simulink model "WMmodel"  (R2025a)
settings: Solver=daessc  StartTime=0.0  StopTime=7200  MaxStep=.5  RelTol=1e-3  AbsTol=1e-3
PreLoadFcn:
  | WMmodel_ini
  | Control_Ts=2;
values from neighbouring files (symbols this model uses):
  inletPipeDia = 0.025    [WMmodel_ini.m]
  motorRatedSpeed = 1250    [WMmodel_ini.m]
  motorRotorInertia = 1e-3    (= 0.001)    [WMmodel_ini.m]
  outerDrumLen = 1    [WMmodel_ini.m]
  outerDrumMaxFill = 50    [WMmodel_ini.m]
  outletPipeDia = 0.025    [WMmodel_ini.m]
  valveSpoolPosMax = 0.01    [WMmodel_ini.m]
libraries: fl_lib x17, nesl_utility x9, SimscapeFluids_lib x7, sdl_lib x1, ee_lib x1
CloseFcn:
  | try,close(h1_sscv_washing_machine_fault_analysis),end
  | clear h1_sscv_washing_machine_fault_analysis
  | 
  | clear outerDrumLiqLevel_ini outerDrumArea
  | clear outerDrumLen outerDrumMaxFill
  | clear outletPipeEffLen outletPipeDia
  | clear inletPipeEffLen inletPipeDia
  | clear valveSpoolPosMax valveSpoolTravel
  | clear valveFaultTime pumpShaftSpeed
  | clear motorPhase motorNumPolePair motorRatedMechPower
  | clear motorRatedSpeed motorRatedRMScurr motorEff
  | clear motorRotorInertia motorRotorDamping
  | clear pumpCapacity pumpHead pumpBrakePower
  | clear Control_Ts
  | clear simlog_sscv_washing_machine_fault_analysis tout
Description:
  | Washing Machine Fault Analysis
settings Model: Creator=The MathWorks, Inc.  LastModifiedBy=DR53SF
settings SolverCC: AutoScaleAbsTol=off  MaxConsecutiveMinStep=5  ZeroCrossAlgorithm=Adaptive  AlgebraicLoopSolver=TrustRegion  MaxZcPerStep=1.0
settings DataIOCC: ReturnWorkspaceOutputs=off
settings OptimizationCC: ReuseModelBlockBuffer=off
settings DebuggingCC: IgnoredZcDiagnostic=none  UnconnectedInputMsg=warning  UnconnectedOutputMsg=warning  UnconnectedLineMsg=warning  SymbolicDimsDataTypeCodeGenerationDiagnostic=none
settings ModelReferenceCC: EnableRefExpFcnMdlSchedulingChecks=on
settings SFSimCC: CustomCodeUndefinedFunction=UseInterfaceOnly
settings RTWCC: GPUComputeCapability=3.5  DLArmComputeVersion=19.05
settings SimscapeCC: SimscapeNominalValues="[{\"value\":\"1\",\"unit\":\"A\"},{\"value\":\"1\",\"unit\":\"bar\"},{\"value\":\"1\",\"unit\":\"cm^2\"},{\"value\":\"1\",\"unit\":\"cm^3/s\"},{\"value\":\"1\",\"unit\":\"kJ/kg\"},{\"value\":\"1\",\"unit\":\"kW\"},{\"value\":\"1\",\"unit\":\"l\"},{\"value\":\"1\",\"unit\":\"N\"},{\"value\":\"1\",\"unit\":\"N*m\"},{\"value\":\"1\",\"unit\":\"V\"},{\"value\":\"1e-2\",\"unit\":\"m\"}]"  SimscapeLogType=all  SimscapeLogSimulationStatistics=on  SimscapeLogName=simlog_sscv_washing_machine_fault_analysis  SimscapeLogDataHistory=100000.0

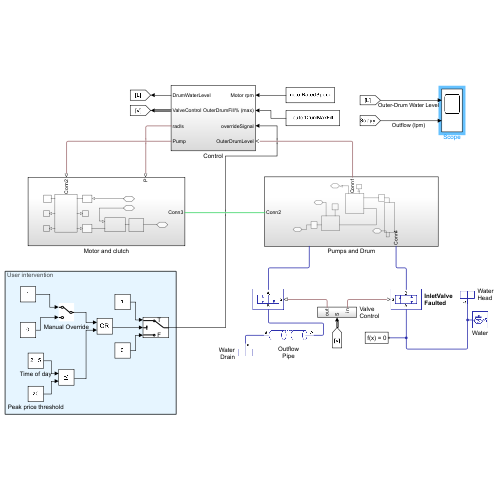
[thumbnail: Simulink's stored preview of the top-level diagram]
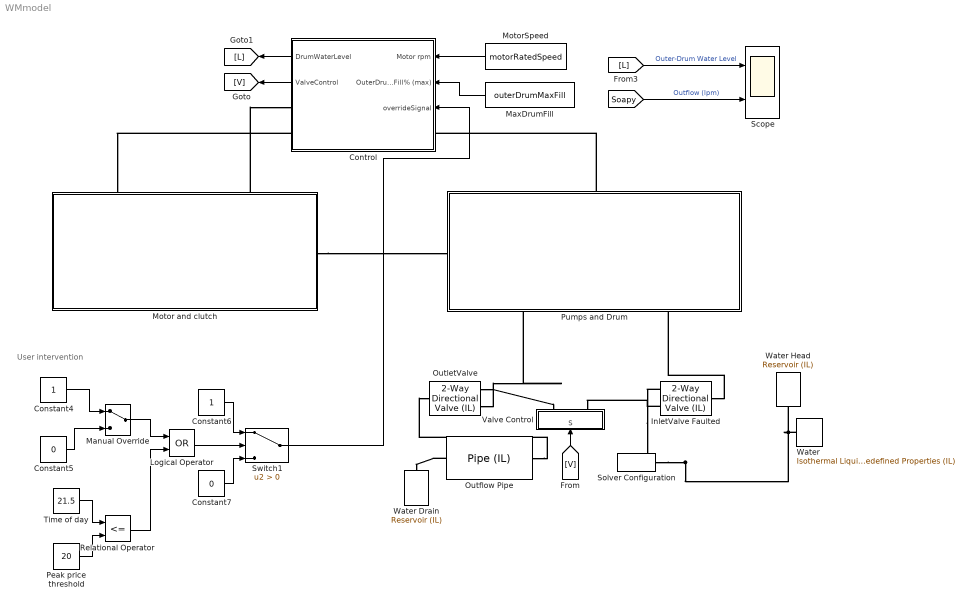
== system WMmodel ==
  note: User intervention
  Constant4 : Constant
  Constant5 : Constant  Value=0
  Constant6 : Constant
  Constant7 : Constant  Value=0
  Control : Subsystem
  InletValve Faulted : SimscapeFluids_lib/Isothermal Liquid/Valves & Orifices/Directional Control Valves/2-Way Directional Valve (IL)  valve_spec=fluids.isothermal_liquid.valves_orifices.directional_control_valves.enum.directional_valve_spec.linear  S_max=valveSpoolPosMax m  del_S_max=valveSpoolTravel m  area_max=(pi/4)*inletPipeDia^2 m^2  area_leak=1e-10 m^2  del_S_TLU=[0, .002, .004, .007, .017] m  orifice_area_TLU=[1e-09, 2.0352e-07, 4.0736e-05, .00011438, .00034356] m^2  del_S_vol_flow_TLU=[0, .002, .004, .007, .017] m  p_diff_TLU=[.003, .05, .7] MPa  vol_flow_TLU=1e-3 * [1.7e-05, 2e-05, 2.6e-05; .0035, .0045, .0053; .7, .9, 1.06; 1.96, 2.5, 3; 6, 7.7, 9.13] m^3/s  Cd=0.64  Re_c=150  smoothing_factor=0.01  pressure_recovery=simscape.enum.onoff.off  area=inf m^2
      settings: InternalSimscapePortConfiguration="{\"Bottom\":[{\"id\":\"B\",\"label\":\"B\",\"type\":\"foundation.isothermal_liquid.isothermal_liquid\"}],\"Left\":[{\"id\":\"S\",\"label\":\"S\",\"type\":\"input\"}],\"Right\":[],\"Top\":[{\"id\":\"A\",\"label\":\"A\",\"type\":\"foundation.isothermal_liquid.isothermal_liquid\"}]}"
  Logical Operator : Logic  Operator=OR  AllPortsSameDT=off  OutDataTypeStr=boolean
  Manual Override : ManualSwitch
  MaxDrumFill : Constant  Value=outerDrumMaxFill  SampleTime=Control_Ts
  Motor and clutch : Subsystem
      settings: PortSchema="{\"entries\":[{\"content\":{\"sides\":[{\"content\":{},\"type\":\"ConnectorPlacement.EquallySpacedRectSide\",\"uuid\":\"2cb3139e-4bf3-4635-b004-e0199a90a34f\"},{\"content\":{\"connectorIds\":[\"RConn1\"],\"side\":\"RIGHT\"},\"type\":\"ConnectorPlacement.EquallySpacedRectSide\",\"uuid\":\"0fa1d438-5e01-49a5-a846-ce380dc8e568\"},{\"content\":{\"connectorIds\":[\"LConn1\",\"LConn2\"],\"side\":\"TOP\"},\"type\":\"ConnectorPlacement.EquallySpacedRectSide\",\"uuid\":\"2360d654-7a91-4e53-9178-c914f2ea5ea3\"}]},\"type\":\"ConnectorPlacement.EquallySpacedConnector\",\"uuid\":\"18350a3b-7253-46c1-a86d-3a50888f0ef8\"}],\"packageUris\":[\"http://schema.mathworks.com/mf0/Connector/R2020b\"],\"version\":\"1.0\"}"
  MotorSpeed : Constant  Value=motorRatedSpeed  SampleTime=Control_Ts
  Outflow Pipe : SimscapeFluids_lib/Isothermal Liquid/Pipes & Fittings/Pipe (IL)  dynamic_compressibility=simscape.enum.onoff.off  inertia=simscape.enum.onoff.off  num_segments=1  pipe_length=outletPipeEffLen m  cross_section_geometry=fluids.isothermal_liquid.pipes_fittings.enum.cross_section_geometry.circular  pipe_diameter=outletPipeDia m  pipe_inner_diameter=0.05 m  pipe_outer_diameter=0.1 m  pipe_width=0.1 m  pipe_height=0.1 m  pipe_major_axis=0.1 m  pipe_minor_axis=0.05 m  pipe_side=0.1 m  pipe_angle=30 deg  pipe_area=0.01 m^2  Dh=0.1128 m  elevation_spec=foundation.enum.constant_variable.constant  elevation_gain=0 m  gravity_spec=foundation.enum.constant_variable.constant  g=9.81 m/s^2  pressure_loss_spec=fluids.isothermal_liquid.pipes_fittings.enum.pressure_loss_spec.haaland  mdot_nominal=[.1, 1] kg/s  p_diff_nominal=[.001, .01] MPa  mdot_threshold=1e-6 kg/s  local_pressure_loss_spec=fluids.isothermal_liquid.pipes_fittings.enum.local_loss_spec.aggregate_length  length_add=1 m  loss_coefficient=0.1  roughness_spec=fluids.isothermal_liquid.pipes_fittings.enum.roughness_spec.commercial_pipe  roughness=15e-6 m  Re_friction_TLU=[400, 1000, 1500, 3000, 4000, 6000, 10000, 20000, 40000, 60000, 100000, 100000000]  friction_factor_TLU=[.264, .112, .071, .0417, .0387, .0268, .025, .0232, .0226, .022, .0214, .0214]  Re_lam=2000  Re_tur=4000  shape_factor=64  pipe_wall_spec=fluids.isothermal_liquid.pipes_fittings.enum.wall_spec.rigid  vol_expansion_spec=fluids.isothermal_liquid.pipes_fittings.enum.vol_expansion_spec.area  area_pressure_gain=1e-6 m^2/MPa  static_pressure_TLU=[.1, 1] MPa  area_pressure_gain_TLU=[1e-05, 1.1e-05] m^2  material_behavior_spec=fluids.isothermal_liquid.pipes_fittings.enum.PipeMaterialBehavior.Linear  diameter_pressure_gain=1e-6 m/MPa  wall_thickness=0.05 m  elastic_modulus=69 GPa  stress_TLU=[276, 310] MPa  strain_TLU=[.004, .02]  stress_assert_action=simscape.enum.assert.action.none  stress_max=400 MPa  poisson_ratio=0.33  wall_time_constant=0.01 s  p0=0.101325 MPa  mdot0=0 kg/s
      settings: InternalSimscapePortConfiguration="{\"Bottom\":[],\"Left\":[{\"id\":\"A\",\"label\":\"A\",\"type\":\"foundation.isothermal_liquid.isothermal_liquid\"}],\"Right\":[{\"id\":\"B\",\"label\":\"B\",\"type\":\"foundation.isothermal_liquid.isothermal_liquid\"}],\"Top\":[]}"
  OutletValve : SimscapeFluids_lib/Isothermal Liquid/Valves & Orifices/Directional Control Valves/2-Way Directional Valve (IL)  valve_spec=fluids.isothermal_liquid.valves_orifices.directional_control_valves.enum.directional_valve_spec.linear  S_max=valveSpoolPosMax m  del_S_max=valveSpoolTravel m  area_max=(pi/4)*outletPipeDia^2 m^2  area_leak=1e-10 m^2  del_S_TLU=[0, .002, .004, .007, .017] m  orifice_area_TLU=[1e-09, 2.0352e-07, 4.0736e-05, .00011438, .00034356] m^2  del_S_vol_flow_TLU=[0, .002, .004, .007, .017] m  p_diff_TLU=[.003, .05, .7] MPa  vol_flow_TLU=1e-3 * [1.7e-05, 2e-05, 2.6e-05; .0035, .0045, .0053; .7, .9, 1.06; 1.96, 2.5, 3; 6, 7.7, 9.13] m^3/s  Cd=0.64  Re_c=150  smoothing_factor=0.01  pressure_recovery=simscape.enum.onoff.off  area=inf m^2
      settings: InternalSimscapePortConfiguration="{\"Bottom\":[{\"id\":\"B\",\"label\":\"B\",\"type\":\"foundation.isothermal_liquid.isothermal_liquid\"}],\"Left\":[{\"id\":\"S\",\"label\":\"S\",\"type\":\"input\"}],\"Right\":[],\"Top\":[{\"id\":\"A\",\"label\":\"A\",\"type\":\"foundation.isothermal_liquid.isothermal_liquid\"}]}"
  Peak price threshold : Constant  Value=20
  Pumps and Drum : Subsystem
      settings: PortSchema="{\"entries\":[{\"content\":{\"sides\":[{\"content\":{\"connectorIds\":[\"LConn1\"]},\"type\":\"ConnectorPlacement.EquallySpacedRectSide\",\"uuid\":\"b631024b-b03a-4ba5-88ab-f74a9126b18e\"},{\"content\":{\"side\":\"RIGHT\"},\"type\":\"ConnectorPlacement.EquallySpacedRectSide\",\"uuid\":\"3fd644d5-b563-41d8-9687-2eeaabd5b41f\"},{\"content\":{\"connectorIds\":[\"LConn2\"],\"side\":\"TOP\"},\"type\":\"ConnectorPlacement.EquallySpacedRectSide\",\"uuid\":\"584c2d8d-6c1b-48df-bb3f-7aaa8986bf0f\"},{\"content\":{\"connectorIds\":[\"RConn1\",\"RConn2\"],\"side\":\"BOTTOM\"},\"type\":\"ConnectorPlacement.EquallySpacedRectSide\",\"uuid\":\"c0a6f7af-5a5a-4250-abd1-d4c5b47363d7\"}]},\"type\":\"ConnectorPlacement.EquallySpacedConnector\",\"uuid\":\"531ac8a9-248c-40a4-8545-6bc81e2e4632\"}],\"packageUris\":[\"http://schema.mathworks.com/mf0/Connector/R2020b\"],\"version\":\"1.0\"}"
  Relational Operator : RelationalOperator  Operator=<=  OutDataTypeStr=boolean  RndMeth=Simplest  InputSameDT=off
  Scope : Scope  NumInputPorts=2
      settings: ActiveDisplayYMinimum=-0.01080540819902244  ActiveDisplayYMaximum=0.56392239287112012  YLabel=Level (m)
  Solver Configuration : nesl_utility/Solver Configuration  PhysicalDomain=network_engine_domain  SubClassName=solver  LeftPortType=input  RightPortType=generic  Tones=[]  Harmonics=[]  SimulateNoise=off  Profile=off  UseLocalSampling=off  EnableSwitchedLinearOptims=on  FrequencyDomain=off  UseCCode=off  RelTol=0.001  AbsTol=1e-06  MinStep=1e-09  ToWorkspace=off  RevertToSquareIcSolve=off  NumHomotopyIterations=100  PhasorMode=off  PhasorModeNumHarmonics=1  ConsistencySolver=NEWTON_FTOL  IndexReductionMethod=DerivativeReplacement  DoDC=off  ResidualTolerance=1e-9  ConsistencyTolSource=GLOBAL  ConsistencyAbsTol=0.001  ConsistencyRelTol=0.001  ConsistencyTolFactor=0.001  UseLocalSolver=off  LocalSolverChoice=NE_BACKWARD_EULER_ADVANCER  ResolveIndetEquations=on  FunctionEvalNumThread=1  LocalSolverSampleTime=.5  DoFixedCost=off  MaxNonlinIter=50  MaxModeIter=2  ComputeImpulses=off  ImpulseIterations=2  LinearAlgebra=auto  LinearAlgebraNumThread=0  EquationFormulation=NE_TIME_EF  DelaysMemoryBudget=1024  AutomaticFiltering=off  FilteringTimeConstant=0.001  PartitionStorageMethod=AS_NEEDED  PartitionMemoryBudget=1024  PartitionMethod=FAST  MultibodyUseLocalSolver=off  MultibodyLocalSolverChoice=ODE1  MultibodyLocalSolverSampleTime=0.001
  Switch1 : Switch  Criteria=u2 > Threshold  SaturateOnIntegerOverflow=off  InputSameDT=off
  Time of day : Constant  Value=21.5
  Valve Control : Subsystem
  Water : SimscapeFluids_lib/Isothermal Liquid/Utilities/Isothermal Liquid Predefined Properties (IL)  fluid_list=fluids.isothermal_liquid.utilities.enum.isothermal_liquid_fluid_list.water  concentration_param_EG=fluids.isothermal_liquid.utilities.enum.isothermal_liquid_concentration.volume_fraction  concentration_param_PG=fluids.isothermal_liquid.utilities.enum.isothermal_liquid_concentration.volume_fraction  c_mass_SW=3.5e-3  c_mass_EG=0.1  c_mass_PG=0.1  c_mass_GL=0.1  c_vol_EG=0.1  c_vol_PG=0.1  beta_L_atm_EG=2.1791 GPa  beta_L_atm_PG=2.1791 GPa  beta_L_atm_GL=2.1791 GPa  p_min_EG=0.01 MPa  p_min_PG=0.01 MPa  p_min_GL=0.01 MPa  T=293.15 K  derate_coeff=1  p_atm=0.101325 MPa  properties_range_check=simscape.enum.assert.action.error  air_fraction=0  polytropic_index=1.0  rho_g_atm=1.225 kg/m^3  air_dissolution_model=simscape.enum.onoff.off  p_crit=3 MPa
      settings: InternalSimscapePortConfiguration="{\"Bottom\":[],\"Left\":[],\"Right\":[{\"id\":\"A\",\"label\":\"\",\"type\":\"foundation.isothermal_liquid.isothermal_liquid\"}],\"Top\":[]}"
  Water Drain : fl_lib/Isothermal Liquid/Elements/Reservoir (IL)  reservoir_type=foundation.enum.constant_controlled.constant  pressure_spec=foundation.enum.pressure_spec.atmospheric  reservoir_pressure=0.101325 MPa
  Water Head : fl_lib/Isothermal Liquid/Elements/Reservoir (IL)  reservoir_type=foundation.enum.constant_controlled.constant  pressure_spec=foundation.enum.pressure_spec.specified  reservoir_pressure=.11 MPa
  wires:
  MaxDrumFill/1 -> Control/2(OuterDrumFill% (max))
  [Soapy] -> Scope/2  "Outflow (lpm)"
  Control/2(ValveControl) -> [V]
  [V] -> Valve Control/1(S)
  MotorSpeed/1 -> Control/1(Motor rpm)
  Control/1(DrumWaterLevel) -> [L]
  [L] -> Scope/1  "Outer-Drum Water Level"
  Constant5/1 -> Manual Override/2
  Constant6/1 -> Switch1/1
  Relational Operator/1 -> Logical Operator/2
  Time of day/1 -> Relational Operator/1
  Constant7/1 -> Switch1/3
  Logical Operator/1 -> Switch1/2
  Manual Override/1 -> Logical Operator/1
  Constant4/1 -> Manual Override/1
  Peak price threshold/1 -> Relational Operator/2
  Switch1/1 -> Control/3(overrideSignal)
  connections:
  Water/RConn1 -- InletValve Faulted/LConn2 -- Solver Configuration/RConn1 -- Water Head/LConn1
  OutletValve/LConn1 -- Valve Control/RConn1
  Outflow Pipe/LConn1 -- OutletValve/RConn1
  Outflow Pipe/RConn1 -- Water Drain/LConn1
  InletValve Faulted/LConn1 -- Valve Control/RConn2
  Motor and clutch/LConn2 -- Control/RConn1
  Control/RConn2 -- Motor and clutch/LConn1
  Pumps and Drum/LConn2 -- Control/LConn1
  Motor and clutch/RConn1 -- Pumps and Drum/LConn1
  OutletValve/LConn2 -- Pumps and Drum/RConn1
  InletValve Faulted/RConn1 -- Pumps and Drum/RConn2

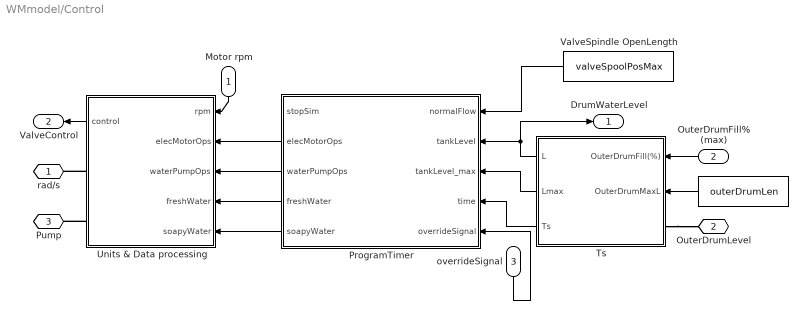
== system WMmodel/Control ==
  Motor rpm : Inport
  OuterDrumFill% (max) : Inport  Port=2
  overrideSignal : Inport  Port=3
  "  " : Constant  Value=outerDrumLen  SampleTime=Control_Ts
  ProgramTimer : MATLAB Function  TreatAsAtomicUnit=on
  Ts : Subsystem
  Units & Data processing : Subsystem
  ValveSpindle OpenLength : Constant  Value=valveSpoolPosMax  SampleTime=Control_Ts
  rad/s : PMIOPort  Side=Right
  OuterDrumLevel : PMIOPort  Port=2  Side=Left
  Pump : PMIOPort  Port=3  Side=Right
  DrumWaterLevel : Outport
  ValveControl : Outport  Port=2
  wires:
  ValveSpindle OpenLength/1 -> ProgramTimer/1(normalFlow)
  ProgramTimer/2(elecMotorOps) -> Units & Data processing/2(elecMotorOps)
  ProgramTimer/3(waterPumpOps) -> Units & Data processing/3(waterPumpOps)
  ProgramTimer/4(freshWater) -> Units & Data processing/4(freshWater)
  ProgramTimer/5(soapyWater) -> Units & Data processing/5(soapyWater)
  Units & Data processing/1(control) -> ValveControl/1
  Motor rpm/1 -> Units & Data processing/1(rpm)
  Ts/1(L) -> ProgramTimer/2(tankLevel), DrumWaterLevel/1
  OuterDrumFill% (max)/1 -> Ts/1(OuterDrumFill(%))
  "  "/1 -> Ts/2(OuterDrumMaxL)
  Ts/2(Lmax) -> ProgramTimer/3(tankLevel_max)
  Ts/3(Ts) -> ProgramTimer/4(time)
  overrideSignal/1 -> ProgramTimer/5(overrideSignal)
  connections:
  Units & Data processing/RConn1 -- rad/s/RConn1
  Units & Data processing/RConn2 -- Pump/RConn1
  Ts/LConn1 -- OuterDrumLevel/RConn1

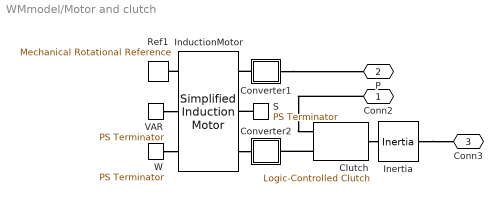
== system WMmodel/Motor and clutch ==
  Clutch : sdl_lib/Clutches/Logic-Controlled Clutch  transition_model=sdl.enum.transitionModel.instant  transition_time_constant=0.1 s  t_friction=10 N*m  t_locked=20 N*m  w_tol=0.001 rad/s  initial_state_locked=sdl.enum.initial_lock.unlocked
      settings: InternalSimscapePortConfiguration="{\"Bottom\":[],\"Left\":[{\"id\":\"E\",\"label\":\"E\",\"type\":\"input\"},{\"id\":\"B\",\"label\":\"B\",\"type\":\"foundation.mechanical.rotational.rotational\"}],\"Right\":[{\"id\":\"F\",\"label\":\"F\",\"type\":\"foundation.mechanical.rotational.rotational\"}],\"Top\":[]}"
  Converter1 : Subsystem
  Converter2 : Subsystem
  InductionMotor : ee_lib/Electromechanical/Asynchronous/Simplified Induction Motor  param=1  R1=1 Ohm  R2=1 Ohm  L1=0.02 H  L2=0.02 H  Lm=0.5 H  P_rated=motorRatedMechPower W  w_mech=motorRatedSpeed rpm  v_rated=230 V  w_rated=50 Hz  i_rated=motorRatedRMScurr A  paramR1=1  E=motorEff  pf=0.93  R1m=1 Ohm  p=motorNumPolePair  n=motorPhase  paramLoad=2  V=230 V  w=50 Hz  J=motorRotorInertia kg*m^2  lam=motorRotorDamping N*m/(rad/s)  speed0=0 rpm  alpha=[.00393, .00393] 1/K  Tmeas=25 degC  thermal_masses=[100, 100] J/K  initial_temperatures=[25, 25] degC
      settings: InternalSimscapePortConfiguration="{\"Bottom\":[],\"Left\":[{\"id\":\"wm\",\"label\":\"wm\",\"type\":\"output\"},{\"id\":\"slip\",\"label\":\"s\",\"type\":\"output\"},{\"id\":\"R\",\"label\":\"R\",\"type\":\"foundation.mechanical.rotational.rotational\"}],\"Right\":[{\"id\":\"Watts\",\"label\":\"W\",\"type\":\"output\"},{\"id\":\"VARs\",\"label\":\"VAR\",\"type\":\"output\"},{\"id\":\"C\",\"label\":\"C\",\"type\":\"foundation.mechanical.rotational.rotational\"}],\"Top\":[]}"
  Inertia : fl_lib/Mechanical/Rotational Elements/Inertia  inertia=0.01 kg*m^2  num_ports=foundation.enum.numPorts2.two  w_specify=off  w_priority=High  w=0 rad/s  w_nominal_specify=off  w_nominal_value=1  w_nominal_unit=rad/s  t_specify=off  t_priority=None  t=0 N*m  t_nominal_specify=off  t_nominal_value=1  t_nominal_unit=N*m
      settings: InternalSimscapePortConfiguration="{\"Bottom\":[],\"Left\":[{\"id\":\"I\",\"label\":\"\",\"type\":\"foundation.mechanical.rotational.rotational\"}],\"Right\":[{\"id\":\"J\",\"label\":\"\",\"type\":\"foundation.mechanical.rotational.rotational\"}],\"Top\":[]}"
  Ref1 : fl_lib/Mechanical/Rotational Elements/Mechanical Rotational Reference
  S : fl_lib/Physical Signals/Sinks/PS Terminator
  "VAR    " : fl_lib/Physical Signals/Sinks/PS Terminator
  W : fl_lib/Physical Signals/Sinks/PS Terminator
  Conn2 : PMIOPort  Side=Left
  P : PMIOPort  Port=2  Side=Left
  Conn3 : PMIOPort  Port=3  Side=Right
  connections:
  Conn2/RConn1 -- Clutch/LConn1
  "VAR    "/LConn1 -- InductionMotor/RConn2
  InductionMotor/RConn3 -- Ref1/LConn1
  InductionMotor/LConn1 -- Converter2/RConn1
  W/LConn1 -- InductionMotor/RConn1
  Clutch/LConn2 -- Converter2/LConn1
  Converter1/RConn1 -- P/RConn1
  Clutch/RConn1 -- Inertia/LConn1
  S/LConn1 -- InductionMotor/LConn2
  Converter1/LConn1 -- InductionMotor/LConn3
  Inertia/RConn1 -- Conn3/RConn1

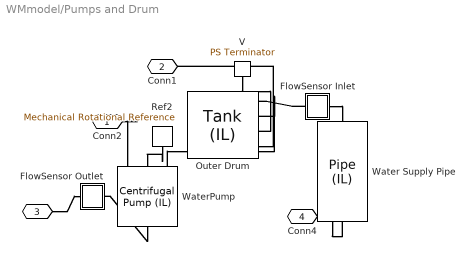
== system WMmodel/Pumps and Drum ==
  FlowSensor Inlet : Subsystem
  FlowSensor Outlet : Subsystem
  Outer Drum : SimscapeFluids_lib/Isothermal Liquid/Tanks & Accumulators/Tank (IL)  num_inlet=fluids.isothermal_liquid.tanks_accumulators.enum.NumInlet.Two  pressure_spec=foundation.enum.pressure_spec.atmospheric  tank_pressure=0.101325 MPa  volume_spec=fluids.isothermal_liquid.tanks_accumulators.enum.TankVolumeSpec.Constant  tank_area=outerDrumArea m^2  level_TLU=[0, 3, 5] m  volume_TLU=[0, 4, 6] m^3  inlet_height_A=0.1 m  inlet_area_A=0.01 m^2  inlet_height_AB=[0, 0] m  inlet_area_AB=[(pi/4)*inletPipeDia^2, (pi/4)*outletPipeDia^2] m^2  inlet_height_ABC=[.1, .05, 0] m  inlet_area_ABC=[.01, .01, .01] m^2  inlet_height_ABCD=linspace(0.1, 0, 4) m  inlet_area_ABCD=0.01 * ones(1, 4) m^2  inlet_height_ABCDE=linspace(0.1, 0, 5) m  inlet_area_ABCDE=0.01 * ones(1, 5) m^2  inlet_height_ABCDEF=linspace(0.1, 0, 6) m  inlet_area_ABCDEF=0.01 * ones(1, 6) m^2  level_check=simscape.enum.assert.action.none  capacity_check=simscape.enum.assert.action.none  max_capacity=10 m^3  g=9.81 m/s^2  level_specify=on  level_priority=High  level=outerDrumLiqLevel_ini m  level_nominal_specify=off  level_nominal_value=1  level_nominal_unit=m  volume_specify=off  volume_priority=High  volume=.5 m^3  volume_nominal_specify=off  volume_nominal_value=1  volume_nominal_unit=m^3  mass_specify=off  mass_priority=None  mass=5e+3 kg  mass_nominal_specify=off  mass_nominal_value=1  mass_nominal_unit=kg
      settings: InternalSimscapePortConfiguration="{\"Bottom\":[],\"Left\":[{\"id\":\"A\",\"label\":\"A\",\"type\":\"foundation.isothermal_liquid.isothermal_liquid\"},{\"id\":\"B\",\"label\":\"B\",\"type\":\"foundation.isothermal_liquid.isothermal_liquid\"}],\"Right\":[],\"Top\":[{\"id\":\"V\",\"label\":\"V\",\"type\":\"output\"},{\"id\":\"L\",\"label\":\"L\",\"type\":\"output\"}]}"
  Ref2 : fl_lib/Mechanical/Rotational Elements/Mechanical Rotational Reference
  V : fl_lib/Physical Signals/Sinks/PS Terminator
  Water Supply Pipe : SimscapeFluids_lib/Isothermal Liquid/Pipes & Fittings/Pipe (IL)  dynamic_compressibility=simscape.enum.onoff.off  inertia=simscape.enum.onoff.off  num_segments=1  pipe_length=inletPipeEffLen m  cross_section_geometry=fluids.isothermal_liquid.pipes_fittings.enum.cross_section_geometry.circular  pipe_diameter=inletPipeDia m  pipe_inner_diameter=0.05 m  pipe_outer_diameter=0.1 m  pipe_width=0.1 m  pipe_height=0.1 m  pipe_major_axis=0.1 m  pipe_minor_axis=0.05 m  pipe_side=0.1 m  pipe_angle=30 deg  pipe_area=0.01 m^2  Dh=0.1128 m  elevation_spec=foundation.enum.constant_variable.constant  elevation_gain=0 m  gravity_spec=foundation.enum.constant_variable.constant  g=9.81 m/s^2  pressure_loss_spec=fluids.isothermal_liquid.pipes_fittings.enum.pressure_loss_spec.haaland  mdot_nominal=[.1, 1] kg/s  p_diff_nominal=[.001, .01] MPa  mdot_threshold=1e-6 kg/s  local_pressure_loss_spec=fluids.isothermal_liquid.pipes_fittings.enum.local_loss_spec.aggregate_length  length_add=1 m  loss_coefficient=0.1  roughness_spec=fluids.isothermal_liquid.pipes_fittings.enum.roughness_spec.commercial_pipe  roughness=15e-6 m  Re_friction_TLU=[400, 1000, 1500, 3000, 4000, 6000, 10000, 20000, 40000, 60000, 100000, 100000000]  friction_factor_TLU=[.264, .112, .071, .0417, .0387, .0268, .025, .0232, .0226, .022, .0214, .0214]  Re_lam=2000  Re_tur=4000  shape_factor=64  pipe_wall_spec=fluids.isothermal_liquid.pipes_fittings.enum.wall_spec.rigid  vol_expansion_spec=fluids.isothermal_liquid.pipes_fittings.enum.vol_expansion_spec.area  area_pressure_gain=1e-6 m^2/MPa  static_pressure_TLU=[.1, 1] MPa  area_pressure_gain_TLU=[1e-05, 1.1e-05] m^2  material_behavior_spec=fluids.isothermal_liquid.pipes_fittings.enum.PipeMaterialBehavior.Linear  diameter_pressure_gain=1e-6 m/MPa  wall_thickness=0.05 m  elastic_modulus=69 GPa  stress_TLU=[276, 310] MPa  strain_TLU=[.004, .02]  stress_assert_action=simscape.enum.assert.action.none  stress_max=400 MPa  poisson_ratio=0.33  wall_time_constant=0.01 s  p0=0.101325 MPa  mdot0=0 kg/s
      settings: InternalSimscapePortConfiguration="{\"Bottom\":[],\"Left\":[{\"id\":\"A\",\"label\":\"A\",\"type\":\"foundation.isothermal_liquid.isothermal_liquid\"}],\"Right\":[{\"id\":\"B\",\"label\":\"B\",\"type\":\"foundation.isothermal_liquid.isothermal_liquid\"}],\"Top\":[]}"
  WaterPump : SimscapeFluids_lib/Isothermal Liquid/Pumps & Motors/Centrifugal Pump (IL)  Tag={'toolbox/physmod/fluids/fluids/SimscapeFluids_lib_parts';'Isothermal_Liquid/Pumps_and_Motors/Centrifugal_Pump__IL_/Grundfos/SP_75S_3Stages.xml'}  pump_parameterization=fluids.isothermal_liquid.pumps_motors.enum.centrifugal_pump_spec.table1D  capacity_ref_nominal=45 lpm  head_ref_nominal=40 m  power_ref_nominal=0.85 kW  head_ref_max=60 m  capacity_ref_max=80 lpm  omega_ref_analytic=1770 rpm  capacity_ref_1D_TLU=pumpCapacity lpm  head_ref_1D_TLU=pumpHead m  power_ref_1D_TLU=pumpBrakePower HP_DIN  omega_ref_1D=pumpShaftSpeed rpm  rho_ref_1D=998.21 % Library default kg/m^3  omega_threshold_factor=1e-2  capacity_2D_TLU=[16.67 23.33 30 40 53.33 60] lpm  omega_2D_TLU=[2450 2800 3150 3500] rpm  head_2D_TLU=[25 32.7 42.5 50;24 31.7 41 49;22.7 30.5 39 47.5;20 28 36 45;15.7 24 32 40;12.5 21 29.5 37.5] m  power_2D_TLU=[0.28 0.38 0.5 0.6;0.31 0.41 0.55 0.68;0.33 0.44 0.6 0.75;0.36 0.48 0.65 0.83;0.38 0.53 0.72 0.93;0.39 0.55 0.75 0.97] kW  rho_ref_2D=998.21 kg/m^3  diameter_ratio=1 % Library default  mech_orientation=fluids.isothermal_liquid.pumps_motors.enum.centrifugal_pump_mech_orientation.positive  operation_check=simscape.enum.assert.action.none
      settings: InternalSimscapePortConfiguration="{\"Bottom\":[{\"id\":\"A\",\"label\":\"A\",\"type\":\"foundation.isothermal_liquid.isothermal_liquid\"}],\"Left\":[],\"Right\":[{\"id\":\"R\",\"label\":\"R\",\"type\":\"foundation.mechanical.rotational.rotational\"},{\"id\":\"C\",\"label\":\"C\",\"type\":\"foundation.mechanical.rotational.rotational\"}],\"Top\":[{\"id\":\"B\",\"label\":\"B\",\"type\":\"foundation.isothermal_liquid.isothermal_liquid\"}]}"
  Conn2 : PMIOPort  Side=Left
  Conn1 : PMIOPort  Port=2  Side=Left
  " " : PMIOPort  Port=3  Side=Right
  Conn4 : PMIOPort  Port=4  Side=Right
  connections:
  Outer Drum/LConn4 -- Conn1/RConn1
  FlowSensor Inlet/RConn1 -- Outer Drum/LConn1
  FlowSensor Inlet/LConn1 -- Water Supply Pipe/RConn1
  Conn4/RConn1 -- Water Supply Pipe/LConn1
  Ref2/LConn1 -- WaterPump/RConn2
  V/LConn1 -- Outer Drum/LConn3
  WaterPump/RConn3 -- Outer Drum/LConn2
  WaterPump/LConn1 -- FlowSensor Outlet/RConn1
  " "/RConn1 -- FlowSensor Outlet/LConn1
  Conn2/RConn1 -- WaterPump/RConn1

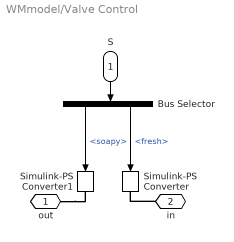
== system WMmodel/Valve Control ==
  S : Inport
  Bus Selector : BusSelector  OutputSignals=fresh,soapy
  Simulink-PS Converter : nesl_utility/Simulink-PS Converter  PhysicalDomain=network_engine_domain  SubClassName=ps_input  LeftPortType=input  RightPortType=output  PseudoPeriodic=off  Frequencies=[]  NoiseDistribution=none  NoiseParameters=[]  Unit=m  AffineConversion=off  FilteringAndDerivatives=filter  SimscapeFilterOrder=1  InputFilterTimeConstant=0.001  UdotUserProvided=0
  Simulink-PS Converter1 : nesl_utility/Simulink-PS Converter  PhysicalDomain=network_engine_domain  SubClassName=ps_input  LeftPortType=input  RightPortType=output  PseudoPeriodic=off  Frequencies=[]  NoiseDistribution=none  NoiseParameters=[]  Unit=m  AffineConversion=off  FilteringAndDerivatives=filter  SimscapeFilterOrder=1  InputFilterTimeConstant=0.001  UdotUserProvided=0
  out : PMIOPort  Side=Right
  in : PMIOPort  Port=2  Side=Right
  wires:
  Bus Selector/1 -> Simulink-PS Converter/1  "<fresh>"
  S/1 -> Bus Selector/1
  Bus Selector/2 -> Simulink-PS Converter1/1  "<soapy>"
  connections:
  in/RConn1 -- Simulink-PS Converter/RConn1
  out/RConn1 -- Simulink-PS Converter1/RConn1

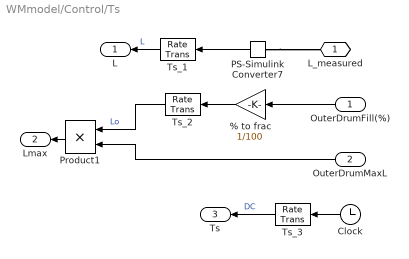
== system WMmodel/Control/Ts ==
  OuterDrumFill(%) : Inport
  OuterDrumMaxL : Inport  Port=2
  % to frac : Gain  Gain=1/100
  Clock : Clock
  PS-Simulink Converter7 : nesl_utility/PS-Simulink Converter  PhysicalDomain=network_engine_domain  SubClassName=ps_output  LeftPortType=input  RightPortType=output  PseudoPeriodic=off  Frequencies=[]  VectorFormat=1-D array  Unit=inherit  AffineConversion=off
  Product1 : Product
  Ts_1 : RateTransition  OutPortSampleTime=Control_Ts
  Ts_2 : RateTransition  OutPortSampleTime=Control_Ts
  Ts_3 : RateTransition  OutPortSampleTime=Control_Ts
  L_measured : PMIOPort  Side=Left
  L : Outport
  Lmax : Outport  Port=2
  Ts : Outport  Port=3
  wires:
  Ts_1/1 -> L/1  "L"
  Product1/1 -> Lmax/1
  Clock/1 -> Ts_3/1
  Ts_3/1 -> Ts/1  "DC"
  Ts_2/1 -> Product1/1  "Lo"
  OuterDrumMaxL/1 -> Product1/2
  OuterDrumFill(%)/1 -> % to frac/1
  PS-Simulink Converter7/1 -> Ts_1/1
  % to frac/1 -> Ts_2/1
  connections:
  PS-Simulink Converter7/LConn1 -- L_measured/RConn1

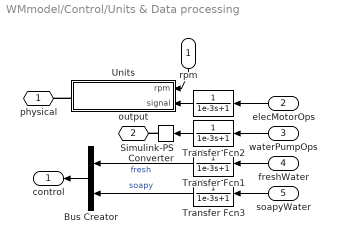
== system WMmodel/Control/Units & Data processing ==
  rpm : Inport
  elecMotorOps : Inport  Port=2
  waterPumpOps : Inport  Port=3
  freshWater : Inport  Port=4
  soapyWater : Inport  Port=5
  " " : TransferFcn  Denominator=[1e-3 1]
  Bus Creator : BusCreator  Inputs=2
  Simulink-PS Converter : nesl_utility/Simulink-PS Converter  PhysicalDomain=network_engine_domain  SubClassName=ps_input  LeftPortType=input  RightPortType=output  PseudoPeriodic=off  Frequencies=[]  NoiseDistribution=none  NoiseParameters=[]  Unit=1  AffineConversion=off  FilteringAndDerivatives=provide  SimscapeFilterOrder=1  InputFilterTimeConstant=0.001  UdotUserProvided=0
  Transfer Fcn1 : TransferFcn  Denominator=[1e-3 1]
  Transfer Fcn2 : TransferFcn  Denominator=[1e-3 1]
  Transfer Fcn3 : TransferFcn  Denominator=[1e-3 1]
  Units : Subsystem
  physical : PMIOPort  Side=Right
  output : PMIOPort  Port=2  Side=Right
  control : Outport
  wires:
  rpm/1 -> Units/1(rpm)
  Bus Creator/1 -> control/1
  elecMotorOps/1 -> " "/1
  soapyWater/1 -> Transfer Fcn3/1
  freshWater/1 -> Transfer Fcn1/1
  Transfer Fcn1/1 -> Bus Creator/1  "fresh"
  Transfer Fcn3/1 -> Bus Creator/2  "soapy"
  Transfer Fcn2/1 -> Simulink-PS Converter/1
  " "/1 -> Units/2(signal)
  waterPumpOps/1 -> Transfer Fcn2/1
  connections:
  Units/RConn1 -- physical/RConn1
  Simulink-PS Converter/RConn1 -- output/RConn1

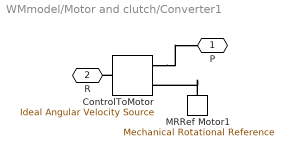
== system WMmodel/Motor and clutch/Converter1 ==
  ControlToMotor : fl_lib/Mechanical/Mechanical Sources/Ideal Angular Velocity Source
  MRRef Motor1 : fl_lib/Mechanical/Rotational Elements/Mechanical Rotational Reference
  P : PMIOPort  Side=Right
  R : PMIOPort  Port=2  Side=Left
  connections:
  ControlToMotor/LConn1 -- R/RConn1
  ControlToMotor/RConn1 -- P/RConn1
  MRRef Motor1/LConn1 -- ControlToMotor/RConn2

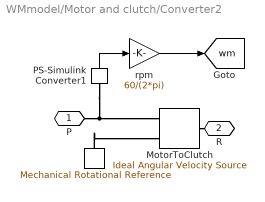
== system WMmodel/Motor and clutch/Converter2 ==
  "      " : fl_lib/Mechanical/Rotational Elements/Mechanical Rotational Reference
  MotorToClutch : fl_lib/Mechanical/Mechanical Sources/Ideal Angular Velocity Source
  PS-Simulink Converter1 : nesl_utility/PS-Simulink Converter  PhysicalDomain=network_engine_domain  SubClassName=ps_output  LeftPortType=input  RightPortType=output  PseudoPeriodic=off  Frequencies=[]  VectorFormat=1-D array  Unit=inherit  AffineConversion=off
  rpm : Gain  Gain=60/(2*pi)
  P : PMIOPort  Side=Right
  R : PMIOPort  Port=2  Side=Left
  tag scope: wm=global
  wires:
  PS-Simulink Converter1/1 -> rpm/1
  rpm/1 -> [wm]
  connections:
  P/RConn1 -- PS-Simulink Converter1/LConn1 -- MotorToClutch/RConn1
  MotorToClutch/LConn1 -- R/RConn1
  "      "/LConn1 -- MotorToClutch/RConn2

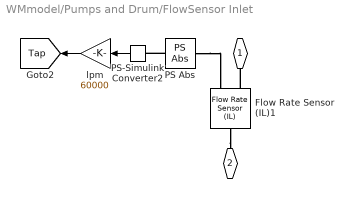
== system WMmodel/Pumps and Drum/FlowSensor Inlet ==
  Flow Rate Sensor (IL)1 : fl_lib/Isothermal Liquid/Sensors/Flow Rate Sensor (IL)  sensor_type=foundation.enum.mass_volumetric_sensor.volumetric
      settings: InternalSimscapePortConfiguration="{\"Bottom\":[],\"Left\":[{\"id\":\"A\",\"label\":\"A\",\"type\":\"foundation.isothermal_liquid.isothermal_liquid\"}],\"Right\":[{\"id\":\"B\",\"label\":\"B\",\"type\":\"foundation.isothermal_liquid.isothermal_liquid\"},{\"id\":\"V\",\"label\":\"V\",\"type\":\"output\"}],\"Top\":[]}"
  PS Abs : fl_lib/Physical Signals/Nonlinear Operators/PS Abs  ZeroCross=true
      settings: InternalSimscapePortConfiguration="{\"Bottom\":[],\"Left\":[{\"id\":\"I\",\"label\":\"\",\"type\":\"input\"}],\"Right\":[{\"id\":\"O\",\"label\":\"\",\"type\":\"output\"}],\"Top\":[]}"
  PS-Simulink Converter2 : nesl_utility/PS-Simulink Converter  PhysicalDomain=network_engine_domain  SubClassName=ps_output  LeftPortType=input  RightPortType=output  PseudoPeriodic=off  Frequencies=[]  VectorFormat=1-D array  Unit=inherit  AffineConversion=off
  lpm : Gain  Gain=60000
  " " : PMIOPort  Side=Right
  "  " : PMIOPort  Port=2  Side=Left
  tag scope: Tap=global
  wires:
  lpm/1 -> [Tap]
  PS-Simulink Converter2/1 -> lpm/1
  connections:
  Flow Rate Sensor (IL)1/RConn1 -- " "/RConn1
  Flow Rate Sensor (IL)1/LConn1 -- "  "/RConn1
  PS Abs/RConn1 -- PS-Simulink Converter2/LConn1
  PS Abs/LConn1 -- Flow Rate Sensor (IL)1/RConn2

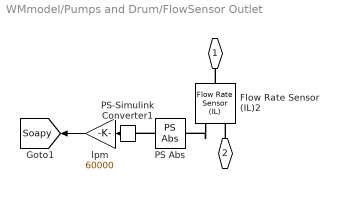
== system WMmodel/Pumps and Drum/FlowSensor Outlet ==
  Flow Rate Sensor (IL)2 : fl_lib/Isothermal Liquid/Sensors/Flow Rate Sensor (IL)  sensor_type=foundation.enum.mass_volumetric_sensor.volumetric
      settings: InternalSimscapePortConfiguration="{\"Bottom\":[],\"Left\":[{\"id\":\"A\",\"label\":\"A\",\"type\":\"foundation.isothermal_liquid.isothermal_liquid\"}],\"Right\":[{\"id\":\"B\",\"label\":\"B\",\"type\":\"foundation.isothermal_liquid.isothermal_liquid\"},{\"id\":\"V\",\"label\":\"V\",\"type\":\"output\"}],\"Top\":[]}"
  PS Abs : fl_lib/Physical Signals/Nonlinear Operators/PS Abs  ZeroCross=true
      settings: InternalSimscapePortConfiguration="{\"Bottom\":[],\"Left\":[{\"id\":\"I\",\"label\":\"\",\"type\":\"input\"}],\"Right\":[{\"id\":\"O\",\"label\":\"\",\"type\":\"output\"}],\"Top\":[]}"
  PS-Simulink Converter1 : nesl_utility/PS-Simulink Converter  PhysicalDomain=network_engine_domain  SubClassName=ps_output  LeftPortType=input  RightPortType=output  PseudoPeriodic=off  Frequencies=[]  VectorFormat=1-D array  Unit=inherit  AffineConversion=off
  lpm : Gain  Gain=60000
  "  " : PMIOPort  Side=Right
  " " : PMIOPort  Port=2  Side=Left
  tag scope: Soapy=global
  wires:
  lpm/1 -> [Soapy]
  PS-Simulink Converter1/1 -> lpm/1
  connections:
  PS Abs/RConn1 -- PS-Simulink Converter1/LConn1
  Flow Rate Sensor (IL)2/RConn2 -- PS Abs/LConn1
  " "/RConn1 -- Flow Rate Sensor (IL)2/RConn1
  Flow Rate Sensor (IL)2/LConn1 -- "  "/RConn1

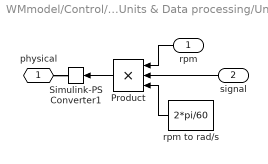
== system WMmodel/Control/Units & Data processing/Units ==
  rpm : Inport
  signal : Inport  Port=2
  Product : Product  Inputs=3
  Simulink-PS Converter1 : nesl_utility/Simulink-PS Converter  PhysicalDomain=network_engine_domain  SubClassName=ps_input  LeftPortType=input  RightPortType=output  PseudoPeriodic=off  Frequencies=[]  NoiseDistribution=none  NoiseParameters=[]  Unit=rad/s  AffineConversion=off  FilteringAndDerivatives=filter  SimscapeFilterOrder=1  InputFilterTimeConstant=0.001  UdotUserProvided=0
  rpm to rad/s : Constant  Value=2*pi/60
  physical : PMIOPort  Side=Right
  wires:
  Product/1 -> Simulink-PS Converter1/1
  rpm/1 -> Product/1
  signal/1 -> Product/2
  rpm to rad/s/1 -> Product/3
  connections:
  physical/RConn1 -- Simulink-PS Converter1/RConn1

== matlab function WMmodel/Control/ProgramTimer ==
  data: normalFlow input; stopSim output; elecMotorOps output; tankLevel input; waterPumpOps output; tankLevel_max input; time input; freshWater output; soapyWater output; overrideSignal input
function [stopSim,elecMotorOps,waterPumpOps,freshWater,soapyWater] = Timer(normalFlow,tankLevel,tankLevel_max,time,overrideSignal)
% -------------------------------------------------------------------------
% INPUTS
    % normalFlow    : Define spool length to allow full flow
    % tankLevel     : Water level in outer drum
    % tankLevel_max : Maximum water level permissible in outer drum
% OUTPUTS
    % stopSim       : End simulation (set to 1) 
    % elecMotorOps  : Set induction motor On (1) or Off (0)
    % waterPumpOps  : Set outlet water pump as On (1) or Off (0)
    % freshWater    : Set spool length of inlet-valve to 'normalFlow' (open)
    %                 or 'leakageFlow' (closed)
    % soapyWater    : Set spool length of outlet-valve to 'normalFlow' (open)
    %                 or 'leakageFlow' (closed)
% -------------------------------------------------------------------------
%
% -------------------------------------------------------------------------
    % Time Operation
    stopSim=0;
    time_min=time/60;
    time_fill=3;
    time_empty=1.8;
    time_rinse=10;
    tankLevel_min=0.05;
    leakageFlow=1e-5; 
    % 1. Fill outer tank with water
    % NEW: OVERRIDE CHECK
    if overrideSignal == 0
        % Force all outputs to a safe, off state
        waterPumpOps=0;
        elecMotorOps=0;
        freshWater=leakageFlow; % Shut inlet valve
        soapyWater=leakageFlow; % Shut outlet valve
        return % Exit the function immediately
    end
    if time_min<=time_fill
        waterPumpOps=0;
        elecMotorOps=0;
        soapyWater=0;
        if tankLevel>tankLevel_max
            freshWater=leakageFlow;
        else
            freshWater=normalFlow; 
        end
    % 2. Mix and rinse
    elseif time_min>time_fill && ...
           time_min<=time_fill+time_rinse
        waterPumpOps=0;
        if tankLevel>1.1*tankLevel_max || tankLevel<0.9*tankLevel_max
            elecMotorOps=0;
        else
            elecMotorOps=1;
        end
        freshWater=leakageFlow; 
        soapyWater=leakageFlow; 
    % 3. Drain soapy water
    elseif time_min>time_fill+time_rinse && ...
           time_min<=time_fill+time_rinse+time_empty
        waterPumpOps=1;
        elecMotorOps=1;
        freshWater=leakageFlow; 
        if tankLevel>tankLevel_min
            soapyWater=normalFlow; 
        else
            soapyWater=leakageFlow;
        end
    % 4. Pull in water again
    elseif time_min>time_fill+time_rinse+time_empty && ...
           time_min<=2*time_fill+time_rinse+time_empty
        waterPumpOps=0;
        elecMotorOps=0;
        soapyWater=0;
        if tankLevel>tankLevel_max
            freshWater=leakageFlow;
        else
            freshWater=normalFlow; 
        end
    % 5. Rinse
    elseif time_min>2*time_fill+time_rinse+time_empty && ...
           time_min<=2*time_fill+2*time_rinse+time_empty
        waterPumpOps=0;
        if tankLevel>1.1*tankLevel_max || tankLevel<0.9*tankLevel_max
            elecMotorOps=0;
        else
            elecMotorOps=1;
        end
        freshWater=leakageFlow; 
        soapyWater=leakageFlow; 
    % 6. Spin and Drain for water
    else
        waterPumpOps=1;    
        elecMotorOps=1;
        freshWater=leakageFlow; 
        if tankLevel>tankLevel_min
            soapyWater=normalFlow; 
        else
            soapyWater=leakageFlow;
            stopSim=1;
        end
    end
%       
end
